simulink model "ProjektAsim"  (R2019b)
settings: Solver=FixedStepAuto  StartTime=0.0  StopTime=10.0  FixedStep=1e-3  RelTol=1e-3
values from neighbouring files (symbols this model uses):
  e = 0.74    [ProjektA.m]
  g = 9.81    [ProjektA.m]
  h = 22    [ProjektA.m]
  v_x = v_0*cosd(alpha)    [ProjektA.m]
  v_y0 = v_0*sind(alpha)    [ProjektA.m]
settings Model: Creator=JH  LastModifiedBy=JH

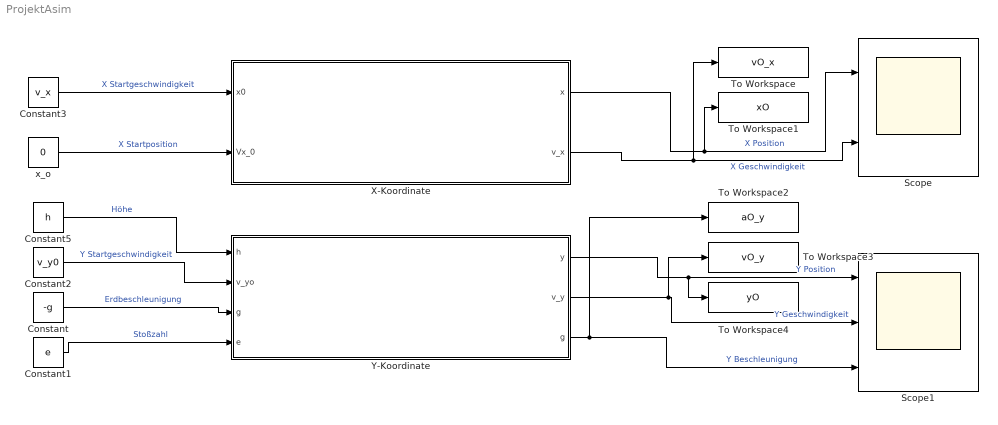
== system ProjektAsim ==
  Constant : Constant  Value=-g
  Constant1 : Constant  Value=e
  Constant2 : Constant  Value=v_y0
  Constant3 : Constant  Value=v_x
  Constant5 : Constant  Value=h
  Scope : Scope  NumInputPorts=2
  Scope1 : Scope  NumInputPorts=3
  To Workspace : ToWorkspace  VariableName=vO_x  SaveFormat=Timeseries  SampleTime=-1
  To Workspace1 : ToWorkspace  VariableName=xO  SaveFormat=Timeseries  SampleTime=-1
  To Workspace2 : ToWorkspace  VariableName=aO_y  SaveFormat=Timeseries  SampleTime=-1
  To Workspace3 : ToWorkspace  VariableName=vO_y  SaveFormat=Timeseries  SampleTime=-1
  To Workspace4 : ToWorkspace  VariableName=yO  SaveFormat=Timeseries  SampleTime=-1
  "X-Koordinate " : Subsystem
  "Y-Koordinate " : Subsystem
  "x_o " : Constant  Value=0
  wires:
  Constant3/1 -> "X-Koordinate "/1(x0)  "X Startgeschwindigkeit"
  Constant2/1 -> "Y-Koordinate "/2("v_yo ")  "Y Startgeschwindigkeit"
  Constant/1 -> "Y-Koordinate "/3(g)  "Erdbeschleunigung"
  Constant1/1 -> "Y-Koordinate "/4(e)  "Stoßzahl"
  "x_o "/1 -> "X-Koordinate "/2("Vx_0 ")  "X Startposition"
  Constant5/1 -> "Y-Koordinate "/1("h ")  "Höhe"
  "Y-Koordinate "/3("g ") -> To Workspace2/1, Scope1/3  "Y Beschleunigung"
  "Y-Koordinate "/2("v_y ") -> To Workspace3/1, Scope1/2  "Y Geschwindigkeit"
  "Y-Koordinate "/1("y ") -> To Workspace4/1, Scope1/1  "Y Position"
  "X-Koordinate "/2("v_x ") -> Scope/2, To Workspace/1  "X Geschwindigkeit"
  "X-Koordinate "/1("x ") -> Scope/1, To Workspace1/1  "X Position"

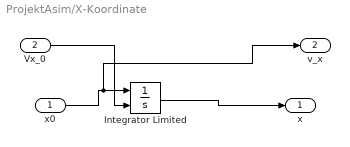
== system ProjektAsim/X-Koordinate  ==
  x0 : Inport
  "Vx_0 " : Inport  Port=2
  Integrator Limited : Integrator  InitialConditionSource=external  LimitOutput=on  LowerSaturationLimit=0
  "x " : Outport
  "v_x " : Outport  Port=2
  wires:
  x0/1 -> "v_x "/1, Integrator Limited/1
  Integrator Limited/1 -> "x "/1
  "Vx_0 "/1 -> Integrator Limited/2

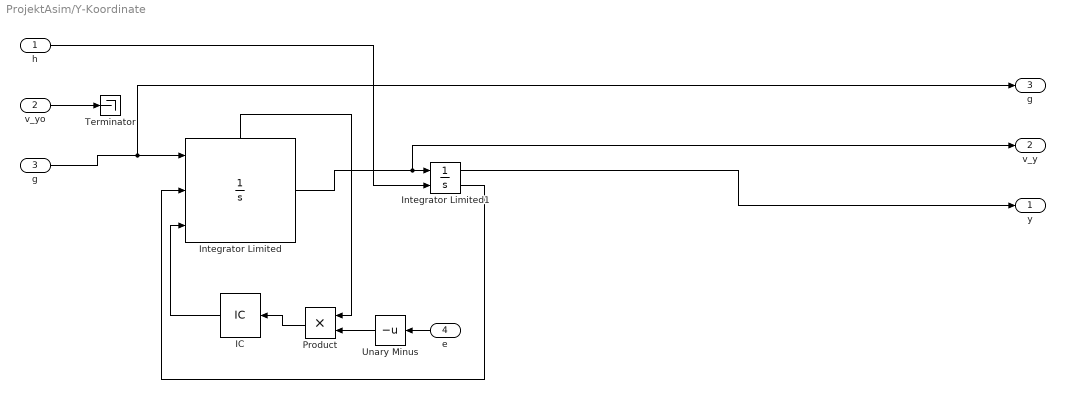
== system ProjektAsim/Y-Koordinate  ==
  "h " : Inport
  "v_yo " : Inport  Port=2
  g : Inport  Port=3
  e : Inport  Port=4
  IC : InitialCondition  Value=v_y0
  Integrator Limited : Integrator  ExternalReset=falling  InitialConditionSource=external  LowerSaturationLimit=0  ShowStatePort=on
  Integrator Limited1 : Integrator  InitialConditionSource=external  LimitOutput=on  LowerSaturationLimit=0  ShowSaturationPort=on
  Product : Product
  Terminator : Terminator
  Unary Minus : UnaryMinus
  "y " : Outport
  "v_y " : Outport  Port=2
  "g " : Outport  Port=3
  wires:
  g/1 -> "g "/1, Integrator Limited/1
  Integrator Limited/1 -> "v_y "/1, Integrator Limited1/1
  "h "/1 -> Integrator Limited1/2
  Integrator Limited1/1 -> "y "/1
  Integrator Limited1/2 -> Integrator Limited/2
  IC/1 -> Integrator Limited/3
  Product/1 -> IC/1
  Integrator Limited/State -> Product/1
  e/1 -> Unary Minus/1
  Unary Minus/1 -> Product/2
  "v_yo "/1 -> Terminator/1
